simulink model "Dynamic_model"  (R2018b)
settings: Solver=VariableStepAuto  StartTime=0.0  StopTime=100  RelTol=1e-3
libraries: simulink x1
settings Model: Creator=knaik  LastModifiedBy=knaik

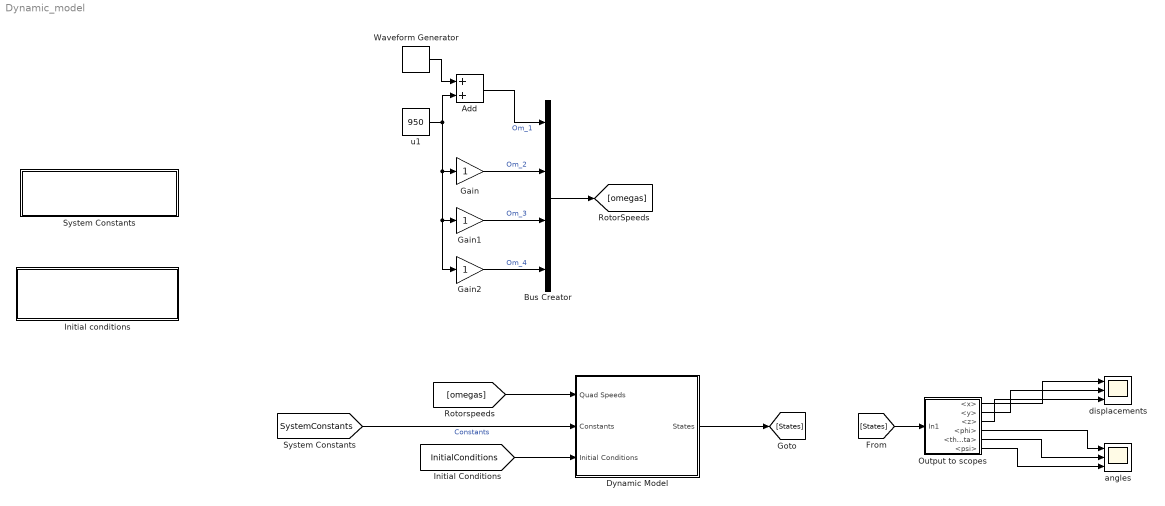
== system Dynamic_model ==
  Add : Sum
  Bus Creator : BusCreator  Inputs=4
  Dynamic Model : Subsystem
  Gain : Gain
  Gain1 : Gain
  Gain2 : Gain
  "Initial conditions " : Subsystem  mask{x0=5, y0=5, z0=5, x0dot=1, y0dot=1, z0dot=1, phi0=0, theta0=0, psi0=0, phi0dot=0, theta0dot=0, psi0dot=0}
      mask prompts: x0 "Initial X position, in meters"; y0 "Initial Y position, in meters"; z0 "Initial Z position, in meters"; x0dot "Initial Velocity in X direction, m/sec"; y0dot "Initial Velocity in Y direction, m/sec"; z0dot "Initial Velocity in Z direction, m/sec"; phi0 "Initial Roll angle, deg"; theta0 "Initial Pitch angle, deg"; psi0 "Initial Yaw angle, deg"; phi0dot "Initial Roll rate, deg/sec"; theta0dot "Initial Pitch rate, deg/sec"; psi0dot "Initial Yaw rate, deg/sec"
      mask Display: disp('Initial conditions')
  "Output to scopes " : Subsystem
  System Constants : Subsystem  mask{m=1, Ixx=0.00485, Iyy=0.00485, Izz=0.0088, k=0.000003, b=0.0000001, Jr=0.000036, l=0.225, Ax=0.25, Ay=0.25, Az=0.25}
      mask prompts: m "Mass [kg]"; Ixx "Quadrotor Moment of Inertia along x axis [kg.m^2]"; Iyy "Quadrotor Moment of Inertia along y axis, in kg [m^2]"; Izz "Quadrotor Moment of Inertia along z axix [kg.m^2]"; k "Lift Constant"; b "Drag factor"; Jr "Rotor Inertia, in kg.m^2"; l "Length from the rotor to the centre of mass, in m"; Ax "Aerodynamic coefficient X [kg/s]"; Ay "Aerodynamic coefficient Y[kg/s]"; Az "Aerodynamic coefficient Z [kg/s]"
      mask Display: disp('system constants')
  Waveform Generator : simulink/Sources/Waveform Generator  OutMin=[]  OutMax=[]  OutDataTypeStr=double  SelectedSignal=1  Signals=sin(0.3, 0.05, 1)  BlockNames=MultiportSwitch_9555ed5536714e2  SampleTime=0.1
      settings: SourceProductName=Simulink
  angles : Scope  NumInputPorts=3
  displacements : Scope  NumInputPorts=3
  u1 : Constant  Value=950
  wires:
  Bus Creator/1 -> [omegas]
  u1/1 -> Gain2/1, Gain1/1, Gain/1, Add/2
  [omegas] -> Dynamic Model/1("Quad Speeds ")
  [SystemConstants] -> Dynamic Model/2(Constants)  "Constants"
  [InitialConditions] -> Dynamic Model/3("Initial Conditions ")
  Dynamic Model/1(States) -> [States]
  [States] -> "Output to scopes "/1(In1)
  "Output to scopes "/1(<x>) -> displacements/1
  "Output to scopes "/2(<y>) -> displacements/2
  "Output to scopes "/3(<z>) -> displacements/3
  "Output to scopes "/4(<phi>) -> angles/1
  "Output to scopes "/5(<theta>) -> angles/2
  "Output to scopes "/6(<psi>) -> angles/3
  Waveform Generator/1 -> Add/1
  Add/1 -> Bus Creator/1  "Om_1"
  Gain/1 -> Bus Creator/2  "Om_2"
  Gain1/1 -> Bus Creator/3  "Om_3"
  Gain2/1 -> Bus Creator/4  "Om_4"

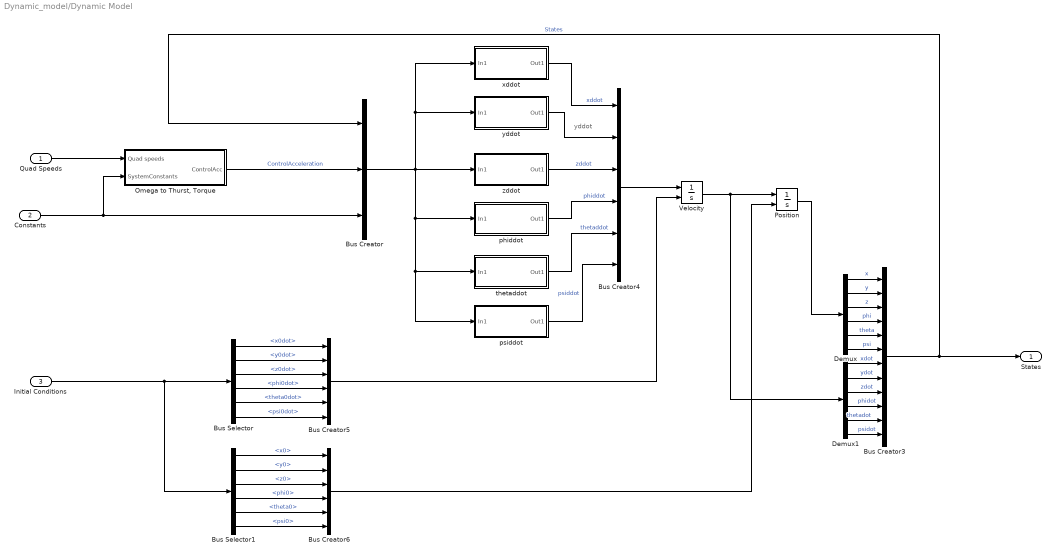
== system Dynamic_model/Dynamic Model ==
  note: yddot
  "Quad Speeds " : Inport
  Constants : Inport  Port=2
  "Initial Conditions " : Inport  Port=3
  Bus Creator : BusCreator  Inputs=3
  Bus Creator3 : BusCreator  Inputs=12
  Bus Creator4 : BusCreator  Inputs=6
  Bus Creator5 : BusCreator  Inputs=6
  Bus Creator6 : BusCreator  Inputs=6
  Bus Selector : BusSelector  OutputSignals=x0dot,y0dot,z0dot,phi0dot,theta0dot,psi0dot
  Bus Selector1 : BusSelector  OutputSignals=x0,y0,z0,phi0,theta0,psi0
  Demux : Demux  Outputs=6
  Demux1 : Demux  Outputs=6
  "Omega to Thurst, Torque" : Subsystem
  Position : Integrator  InitialConditionSource=external
  Velocity : Integrator  InitialConditionSource=external
  phiddot : Subsystem
  psiddot : Subsystem
  thetaddot : Subsystem
  xddot : Subsystem
  yddot : Subsystem
  zddot : Subsystem
  States : Outport
  wires:
  Demux1/1 -> Bus Creator3/7  "xdot"
  Bus Selector1/6 -> Bus Creator6/6  "<psi0>"
  Demux/5 -> Bus Creator3/5  "theta"
  Demux1/6 -> Bus Creator3/12  "psidot"
  Demux/4 -> Bus Creator3/4  "phi"
  Bus Creator/1 -> xddot/1(In1), yddot/1(In1), zddot/1(In1), phiddot/1(In1), thetaddot/1(In1), psiddot/1(In1)
  Constants/1 -> Bus Creator/3, "Omega to Thurst, Torque"/2(SystemConstants)
  Bus Selector1/2 -> Bus Creator6/2  "<y0>"
  Demux/2 -> Bus Creator3/2  "y"
  Demux1/2 -> Bus Creator3/8  "ydot"
  Demux1/5 -> Bus Creator3/11  "thetadot"
  "Omega to Thurst, Torque"/1(ControlAcc) -> Bus Creator/2  "ControlAcceleration"
  Bus Selector1/1 -> Bus Creator6/1  "<x0>"
  Bus Selector1/5 -> Bus Creator6/5  "<theta0>"
  Bus Selector/5 -> Bus Creator5/5  "<theta0dot>"
  "Quad Speeds "/1 -> "Omega to Thurst, Torque"/1("Quad speeds ")
  Demux/6 -> Bus Creator3/6  "psi"
  Bus Selector/6 -> Bus Creator5/6  "<psi0dot>"
  Bus Selector/2 -> Bus Creator5/2  "<y0dot>"
  Velocity/1 -> Position/1, Demux1/1
  zddot/1(Out1) -> Bus Creator4/3  "zddot"
  Bus Creator3/1 -> States/1, Bus Creator/1  "States"
  Demux1/4 -> Bus Creator3/10  "phidot"
  Bus Creator6/1 -> Position/2
  Bus Creator5/1 -> Velocity/2
  Bus Selector/1 -> Bus Creator5/1  "<x0dot>"
  Bus Selector/3 -> Bus Creator5/3  "<z0dot>"
  Demux1/3 -> Bus Creator3/9  "zdot"
  Bus Creator4/1 -> Velocity/1
  Demux/3 -> Bus Creator3/3  "z"
  Bus Selector1/4 -> Bus Creator6/4  "<phi0>"
  Bus Selector/4 -> Bus Creator5/4  "<phi0dot>"
  Bus Selector1/3 -> Bus Creator6/3  "<z0>"
  yddot/1(Out1) -> Bus Creator4/2
  thetaddot/1(Out1) -> Bus Creator4/5  "thetaddot"
  "Initial Conditions "/1 -> Bus Selector/1, Bus Selector1/1
  phiddot/1(Out1) -> Bus Creator4/4  "phiddot"
  xddot/1(Out1) -> Bus Creator4/1  "xddot"
  Position/1 -> Demux/1
  Demux/1 -> Bus Creator3/1  "x"
  psiddot/1(Out1) -> Bus Creator4/6  "psiddot"

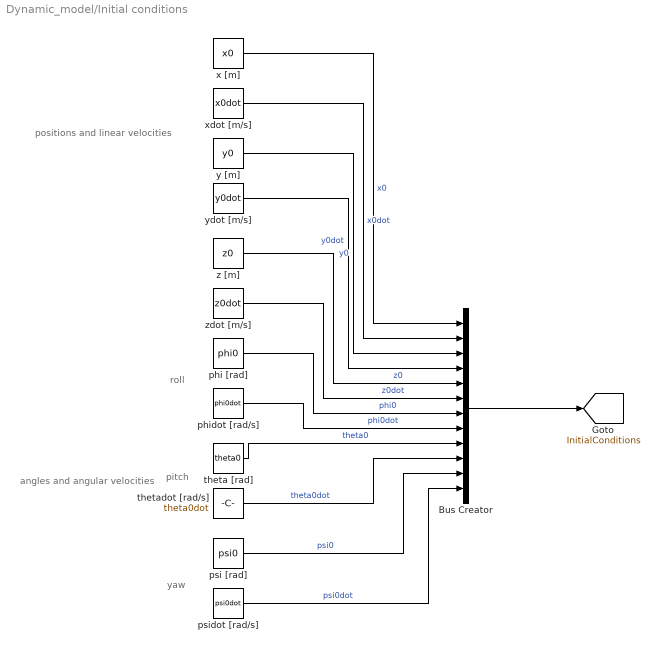
== system Dynamic_model/Initial conditions  ==
  note: positions and linear velocities
  note: angles and angular velocities
  note: yaw
  note: pitch
  note: roll
  Bus Creator : BusCreator  Inputs=12
  phi [rad] : Constant  Value=phi0
  phidot [rad/s] : Constant  Value=phi0dot
  psi [rad] : Constant  Value=psi0
  psidot [rad/s] : Constant  Value=psi0dot
  theta [rad] : Constant  Value=theta0
  thetadot [rad/s] : Constant  Value=theta0dot
  x [m] : Constant  Value=x0
  xdot [m/s] : Constant  Value=x0dot
  y [m] : Constant  Value=y0
  ydot [m/s] : Constant  Value=y0dot
  z [m] : Constant  Value=z0
  zdot [m/s] : Constant  Value=z0dot
  tag scope: InitialConditions=global
  wires:
  x [m]/1 -> Bus Creator/1  "x0"
  xdot [m/s]/1 -> Bus Creator/2  "x0dot"
  y [m]/1 -> Bus Creator/3  "y0"
  ydot [m/s]/1 -> Bus Creator/4  "y0dot"
  z [m]/1 -> Bus Creator/5  "z0"
  zdot [m/s]/1 -> Bus Creator/6  "z0dot"
  phi [rad]/1 -> Bus Creator/7  "phi0"
  phidot [rad/s]/1 -> Bus Creator/8  "phi0dot"
  theta [rad]/1 -> Bus Creator/9  "theta0"
  thetadot [rad/s]/1 -> Bus Creator/10  "theta0dot"
  psi [rad]/1 -> Bus Creator/11  "psi0"
  psidot [rad/s]/1 -> Bus Creator/12  "psi0dot"
  Bus Creator/1 -> [InitialConditions]

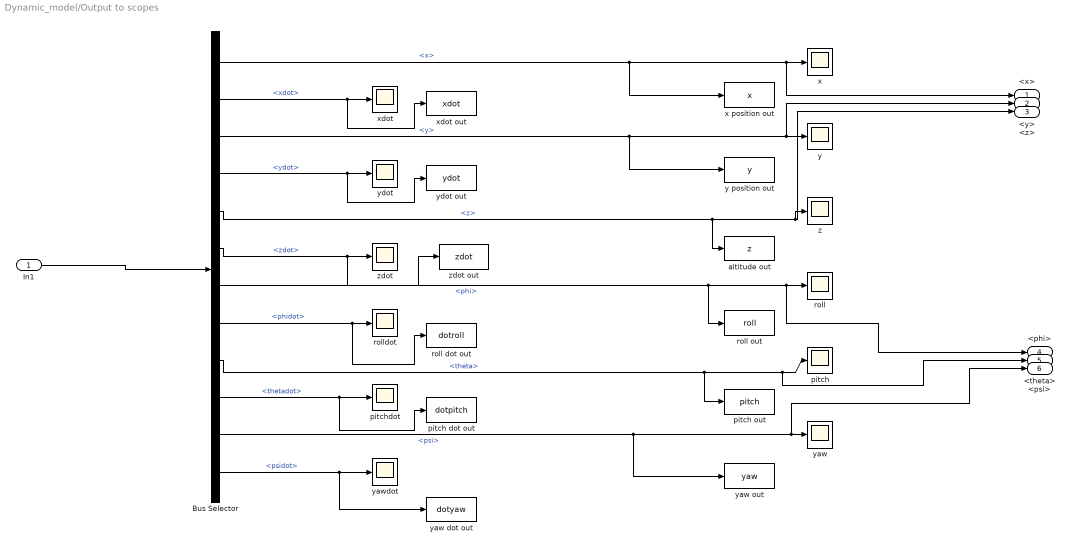
== system Dynamic_model/Output to scopes  ==
  In1 : Inport
  Bus Selector : BusSelector  OutputSignals=x,xdot,y,ydot,z,zdot,phi,phidot,theta,thetadot,psi,psidot
  altitude out : ToWorkspace  VariableName=z  SampleTime=-1
  pitch : Scope
  pitch dot out : ToWorkspace  VariableName=dotpitch  SampleTime=-1
  pitch out : ToWorkspace  VariableName=pitch  SampleTime=-1
  pitchdot : Scope
  roll : Scope
  roll dot out : ToWorkspace  VariableName=dotroll  SampleTime=-1
  roll out : ToWorkspace  VariableName=roll  SampleTime=-1
  rolldot : Scope
  x : Scope
  x position out : ToWorkspace  VariableName=x  SampleTime=-1
  xdot : Scope
  xdot out : ToWorkspace  VariableName=xdot  SampleTime=-1
  y : Scope
  y position out : ToWorkspace  VariableName=y  SampleTime=-1
  yaw : Scope
  yaw dot out : ToWorkspace  VariableName=dotyaw  SampleTime=-1
  yaw out : ToWorkspace  VariableName=yaw  SampleTime=-1
  yawdot : Scope
  ydot : Scope
  ydot out : ToWorkspace  VariableName=ydot  SampleTime=-1
  z : Scope
  zdot : Scope
  zdot out : ToWorkspace  VariableName=zdot  SampleTime=-1
  <x> : Outport
  <y> : Outport  Port=2
  <z> : Outport  Port=3
  <phi> : Outport  Port=4
  <theta> : Outport  Port=5
  <psi> : Outport  Port=6
  wires:
  Bus Selector/5 -> altitude out/1, <z>/1, z/1  "<z>"
  Bus Selector/12 -> yawdot/1, yaw dot out/1  "<psidot>"
  Bus Selector/4 -> ydot/1, ydot out/1  "<ydot>"
  Bus Selector/9 -> pitch out/1, <theta>/1, pitch/1  "<theta>"
  Bus Selector/11 -> yaw out/1, <psi>/1, yaw/1  "<psi>"
  In1/1 -> Bus Selector/1
  Bus Selector/7 -> roll out/1, <phi>/1, roll/1  "<phi>"
  Bus Selector/2 -> xdot/1, xdot out/1  "<xdot>"
  Bus Selector/6 -> zdot/1, zdot out/1  "<zdot>"
  Bus Selector/10 -> pitchdot/1, pitch dot out/1  "<thetadot>"
  Bus Selector/8 -> rolldot/1, roll dot out/1  "<phidot>"
  Bus Selector/1 -> x position out/1, <x>/1, x/1  "<x>"
  Bus Selector/3 -> y position out/1, <y>/1, y/1  "<y>"

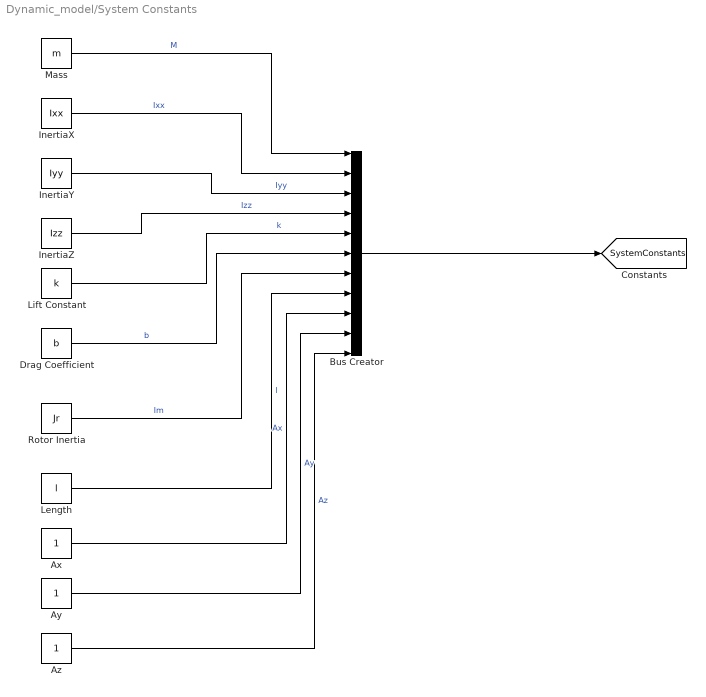
== system Dynamic_model/System Constants ==
  " Mass" : Constant  Value=m
  Ax : Constant
  Ay : Constant
  Az : Constant
  Bus Creator : BusCreator  Inputs=11
  Drag Coefficient : Constant  Value=b
  InertiaX : Constant  Value=Ixx
  InertiaY : Constant  Value=Iyy
  InertiaZ : Constant  Value=Izz
  Length : Constant  Value=l
  Lift Constant : Constant  Value=k
  Rotor Inertia : Constant  Value=Jr
  tag scope: SystemConstants=global
  wires:
  Bus Creator/1 -> [SystemConstants]
  " Mass"/1 -> Bus Creator/1  "M"
  InertiaX/1 -> Bus Creator/2  "Ixx"
  InertiaY/1 -> Bus Creator/3  "Iyy"
  InertiaZ/1 -> Bus Creator/4  "Izz"
  Lift Constant/1 -> Bus Creator/5  "k"
  Drag Coefficient/1 -> Bus Creator/6  "b"
  Rotor Inertia/1 -> Bus Creator/7  "Im"
  Length/1 -> Bus Creator/8  "l"
  Ax/1 -> Bus Creator/9  "Ax"
  Ay/1 -> Bus Creator/10  "Ay"
  Az/1 -> Bus Creator/11  "Az"

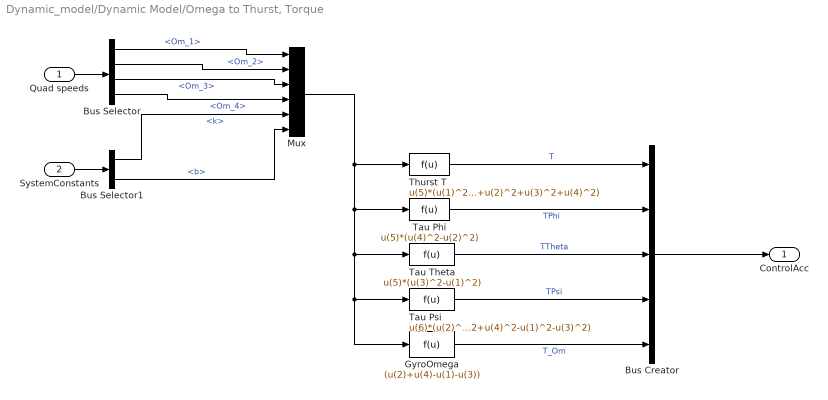
== system Dynamic_model/Dynamic Model/Omega to Thurst, Torque ==
  "Quad speeds " : Inport
  SystemConstants : Inport  Port=2
  Bus Creator : BusCreator  Inputs=5
  Bus Selector : BusSelector  OutputSignals=Om_1,Om_2,Om_3,Om_4
  Bus Selector1 : BusSelector  OutputSignals=k,b
  "GyroOmega " : Fcn  Expr=(u(2)+u(4)-u(1)-u(3))
  Mux : Mux  Inputs=6
  Tau Phi : Fcn  Expr=u(5)*(u(4)^2-u(2)^2)
  Tau Psi : Fcn  Expr=u(6)*(u(2)^2+u(4)^2-u(1)^2-u(3)^2)
  "Tau Theta " : Fcn  Expr=u(5)*(u(3)^2-u(1)^2)
  Thurst T : Fcn  Expr=u(5)*(u(1)^2+u(2)^2+u(3)^2+u(4)^2)
  ControlAcc : Outport
  wires:
  "Quad speeds "/1 -> Bus Selector/1
  SystemConstants/1 -> Bus Selector1/1
  Bus Selector/1 -> Mux/1  "<Om_1>"
  Bus Selector/2 -> Mux/2  "<Om_2>"
  Bus Selector/3 -> Mux/3  "<Om_3>"
  Bus Selector/4 -> Mux/4  "<Om_4>"
  Bus Selector1/1 -> Mux/5  "<k>"
  Bus Selector1/2 -> Mux/6  "<b>"
  Mux/1 -> Thurst T/1, Tau Phi/1, "Tau Theta "/1, Tau Psi/1, "GyroOmega "/1
  Thurst T/1 -> Bus Creator/1  "T"
  Tau Phi/1 -> Bus Creator/2  "TPhi"
  "Tau Theta "/1 -> Bus Creator/3  "TTheta"
  Tau Psi/1 -> Bus Creator/4  "TPsi"
  "GyroOmega "/1 -> Bus Creator/5  "T_Om"
  Bus Creator/1 -> ControlAcc/1

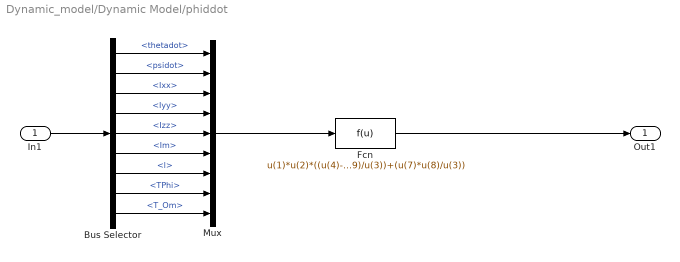
== system Dynamic_model/Dynamic Model/phiddot ==
  In1 : Inport
  Bus Selector : BusSelector  OutputSignals=States.thetadot,States.psidot,Constants.Ixx,Constants.Iyy,Constants.Izz,Constants.Im,Constants.l,ControlAcceleration.TPhi,ControlAcceleration.T_Om
  Fcn : Fcn  Expr=u(1)*u(2)*((u(4)-u(5))/u(3))-(u(6)*u(1)*u(9)/u(3))+(u(7)*u(8)/u(3))
  Mux : Mux  Inputs=9
  Out1 : Outport
  wires:
  Fcn/1 -> Out1/1
  Mux/1 -> Fcn/1
  In1/1 -> Bus Selector/1
  Bus Selector/3 -> Mux/3  "<Ixx>"
  Bus Selector/4 -> Mux/4  "<Iyy>"
  Bus Selector/5 -> Mux/5  "<Izz>"
  Bus Selector/6 -> Mux/6  "<Im>"
  Bus Selector/7 -> Mux/7  "<l>"
  Bus Selector/8 -> Mux/8  "<TPhi>"
  Bus Selector/9 -> Mux/9  "<T_Om>"
  Bus Selector/2 -> Mux/2  "<psidot>"
  Bus Selector/1 -> Mux/1  "<thetadot>"

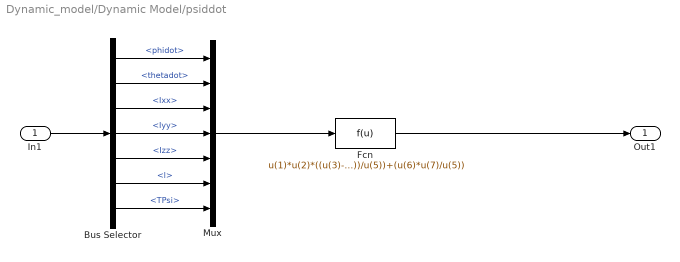
== system Dynamic_model/Dynamic Model/psiddot ==
  In1 : Inport
  Bus Selector : BusSelector  OutputSignals=States.phidot,States.thetadot,Constants.Ixx,Constants.Iyy,Constants.Izz,Constants.l,ControlAcceleration.TPsi
  Fcn : Fcn  Expr=u(1)*u(2)*((u(3)-u(4))/u(5))+(u(6)*u(7)/u(5))
  Mux : Mux  Inputs=7
  Out1 : Outport
  wires:
  Fcn/1 -> Out1/1
  Mux/1 -> Fcn/1
  In1/1 -> Bus Selector/1
  Bus Selector/1 -> Mux/1  "<phidot>"
  Bus Selector/2 -> Mux/2  "<thetadot>"
  Bus Selector/3 -> Mux/3  "<Ixx>"
  Bus Selector/4 -> Mux/4  "<Iyy>"
  Bus Selector/5 -> Mux/5  "<Izz>"
  Bus Selector/6 -> Mux/6  "<l>"
  Bus Selector/7 -> Mux/7  "<TPsi>"

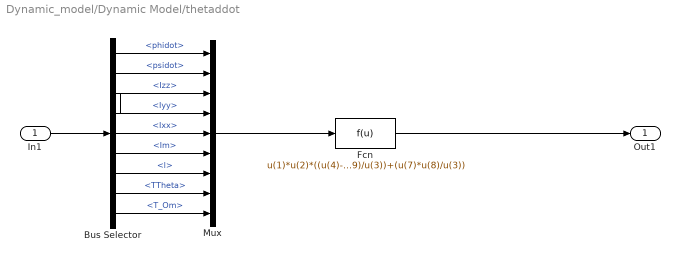
== system Dynamic_model/Dynamic Model/thetaddot ==
  In1 : Inport
  Bus Selector : BusSelector  OutputSignals=States.phidot,States.psidot,Constants.Iyy,Constants.Izz,Constants.Ixx,Constants.Im,Constants.l,ControlAcceleration.TTheta,ControlAcceleration.T_Om
  Fcn : Fcn  Expr=u(1)*u(2)*((u(4)-u(5))/u(3))+(u(6)*u(1)*u(9)/u(3))+(u(7)*u(8)/u(3))
  Mux : Mux  Inputs=9
  Out1 : Outport
  wires:
  Bus Selector/1 -> Mux/1  "<phidot>"
  Bus Selector/2 -> Mux/2  "<psidot>"
  Bus Selector/9 -> Mux/9  "<T_Om>"
  Bus Selector/8 -> Mux/8  "<TTheta>"
  Bus Selector/7 -> Mux/7  "<l>"
  Bus Selector/6 -> Mux/6  "<Im>"
  Bus Selector/3 -> Mux/4  "<Iyy>"
  In1/1 -> Bus Selector/1
  Mux/1 -> Fcn/1
  Fcn/1 -> Out1/1
  Bus Selector/4 -> Mux/3  "<Izz>"
  Bus Selector/5 -> Mux/5  "<Ixx>"

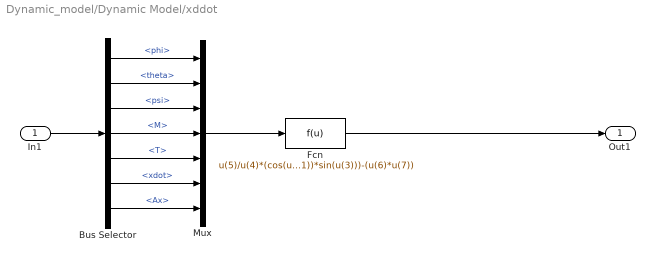
== system Dynamic_model/Dynamic Model/xddot ==
  In1 : Inport
  Bus Selector : BusSelector  OutputSignals=States.phi,States.theta,States.psi,Constants.M,ControlAcceleration.T,States.xdot,Constants.Ax
  Fcn : Fcn  Expr=u(5)/u(4)*(cos(u(1))*sin(u(2))*cos(u(3))+sin(u(1))*sin(u(3)))-(u(6)*u(7))
  Mux : Mux  Inputs=7
  Out1 : Outport
  wires:
  In1/1 -> Bus Selector/1
  Bus Selector/1 -> Mux/1  "<phi>"
  Bus Selector/2 -> Mux/2  "<theta>"
  Bus Selector/3 -> Mux/3  "<psi>"
  Bus Selector/4 -> Mux/4  "<M>"
  Bus Selector/5 -> Mux/5  "<T>"
  Mux/1 -> Fcn/1
  Fcn/1 -> Out1/1
  Bus Selector/6 -> Mux/6  "<xdot>"
  Bus Selector/7 -> Mux/7  "<Ax>"

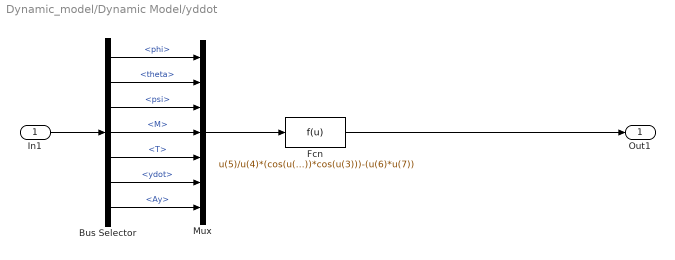
== system Dynamic_model/Dynamic Model/yddot ==
  In1 : Inport
  Bus Selector : BusSelector  OutputSignals=States.phi,States.theta,States.psi,Constants.M,ControlAcceleration.T,States.ydot,Constants.Ay
  Fcn : Fcn  Expr=u(5)/u(4)*(cos(u(1))*sin(u(2))*sin(u(3))-sin(u(1))*cos(u(3)))-(u(6)*u(7))
  Mux : Mux  Inputs=7
  Out1 : Outport
  wires:
  Fcn/1 -> Out1/1
  Mux/1 -> Fcn/1
  Bus Selector/5 -> Mux/5  "<T>"
  Bus Selector/4 -> Mux/4  "<M>"
  Bus Selector/3 -> Mux/3  "<psi>"
  Bus Selector/2 -> Mux/2  "<theta>"
  Bus Selector/1 -> Mux/1  "<phi>"
  In1/1 -> Bus Selector/1
  Bus Selector/6 -> Mux/6  "<ydot>"
  Bus Selector/7 -> Mux/7  "<Ay>"

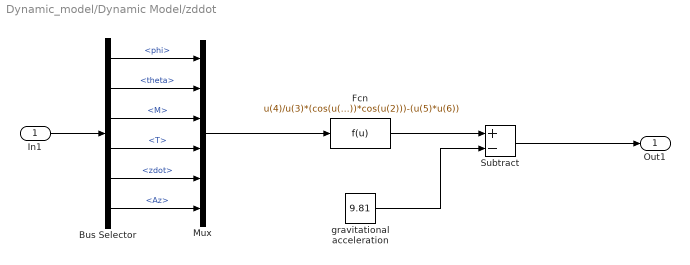
== system Dynamic_model/Dynamic Model/zddot ==
  In1 : Inport
  Bus Selector : BusSelector  OutputSignals=States.phi,States.theta,Constants.M,ControlAcceleration.T,States.zdot,Constants.Az
  Fcn : Fcn  Expr=u(4)/u(3)*(cos(u(1))*cos(u(2)))-(u(5)*u(6))
  Mux : Mux  Inputs=6
  Subtract : Sum  Inputs=+-
  gravitational acceleration : Constant  Value=9.81
  Out1 : Outport
  wires:
  In1/1 -> Bus Selector/1
  Bus Selector/1 -> Mux/1  "<phi>"
  Bus Selector/2 -> Mux/2  "<theta>"
  Mux/1 -> Fcn/1
  Bus Selector/3 -> Mux/3  "<M>"
  Bus Selector/4 -> Mux/4  "<T>"
  Fcn/1 -> Subtract/1
  gravitational acceleration/1 -> Subtract/2
  Subtract/1 -> Out1/1
  Bus Selector/5 -> Mux/5  "<zdot>"
  Bus Selector/6 -> Mux/6  "<Az>"
